simulink model "bldc"  (R2022a)
settings: Solver=VariableStepAuto  StartTime=0.0  StopTime=60  FixedStep=0.0001  MaxStep=0.01  RelTol=1e-3
model workspace (MAT data in the model file):
  gPWM_U_ptr : handle (value not decoded)
  gPWM_V_ptr : handle (value not decoded)
  gPWM_W_ptr : handle (value not decoded)
values from neighbouring files (symbols this model uses):
  D = 0.00075    [init_bldc.m]
  J = 0.00025    [init_bldc.m]
  Ld = 0.0009447    [init_bldc.m]
  Lq = 0.0009447    [init_bldc.m]
  P = 7    [init_bldc.m]
  qsi = 0.006198    [init_bldc.m]
  R = 0.453    [init_bldc.m]
  V = 24    [init_bldc.m]
settings Model: Creator=sshio  LastModifiedBy=sshio
settings DebuggingCC: UnconnectedInputMsg=warning  UnconnectedOutputMsg=warning  UnconnectedLineMsg=warning
settings RTWCC: DLArmComputeVersion=19.05

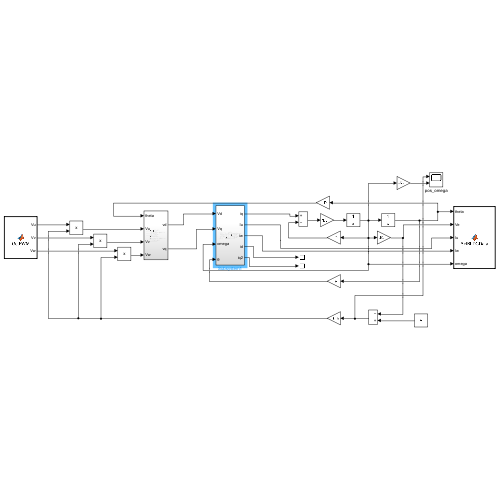
[thumbnail: Simulink's stored preview of the top-level diagram]
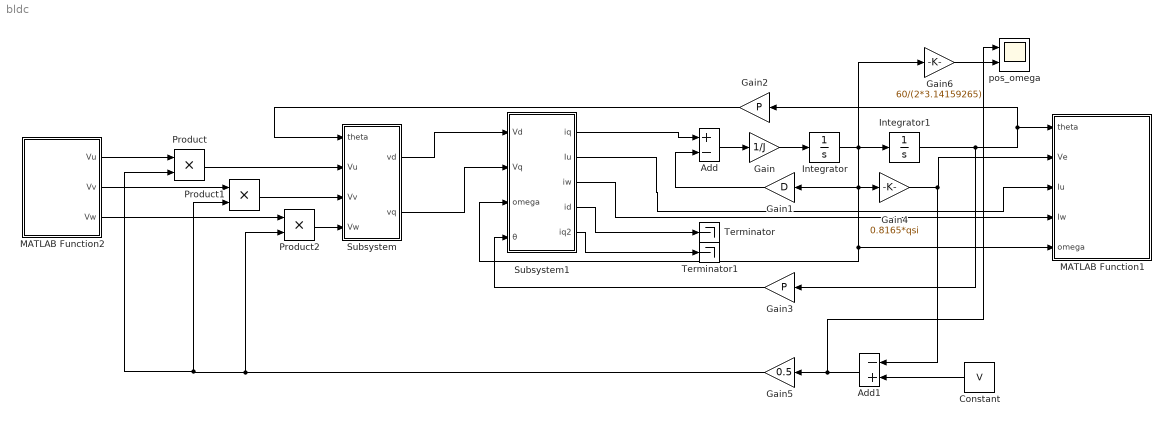
== system bldc ==
  Add : Sum  Inputs=+-
  Add1 : Sum  Inputs=-+
  Constant : Constant  Value=V
  Gain : Gain  Gain=1/J
  Gain1 : Gain  Gain=D
  Gain2 : Gain  Gain=P
  Gain3 : Gain  Gain=P
  Gain4 : Gain  Gain=0.8165*qsi
  Gain5 : Gain  Gain=0.5
  Gain6 : Gain  Gain=60/(2*3.14159265)
  Integrator : Integrator
  Integrator1 : Integrator
  MATLAB Function1 : MATLAB Function  TreatAsAtomicUnit=on  SystemSampleTime=0.0001
  MATLAB Function2 : MATLAB Function  TreatAsAtomicUnit=on  SystemSampleTime=0.0001
  Product : Product
  Product1 : Product
  Product2 : Product
  Subsystem : Subsystem
  Subsystem1 : Subsystem
  Terminator : Terminator
  Terminator1 : Terminator
  pos_omega : Scope  NumInputPorts=2
  wires:
  Subsystem/2(vq) -> Subsystem1/2(Vq)
  Integrator/1 -> Gain6/1, Integrator1/1, Gain4/1, Gain1/1, MATLAB Function1/5(omega), Subsystem1/3(omega)
  Gain/1 -> Integrator/1
  Add/1 -> Gain/1
  Subsystem1/1(iq) -> Add/1
  Gain1/1 -> Add/2
  Gain2/1 -> Subsystem/1(theta)
  Gain3/1 -> Subsystem1/4(θ)
  Subsystem1/3(iw) -> MATLAB Function1/4(Iw)
  Gain4/1 -> Add1/1, MATLAB Function1/2(Ve)
  Constant/1 -> Add1/2
  Gain5/1 -> Product/2, Product1/2, Product2/2
  Product2/1 -> Subsystem/4(Vw)
  MATLAB Function2/2(Vv) -> Product1/1
  MATLAB Function2/3(Vw) -> Product2/1
  Product1/1 -> Subsystem/3(Vv)
  Product/1 -> Subsystem/2(Vu)
  MATLAB Function2/1(Vu) -> Product/1
  Integrator1/1 -> Gain3/1, Gain2/1, MATLAB Function1/1(theta)
  Subsystem1/2(Iu) -> MATLAB Function1/3(Iu)
  Add1/1 -> pos_omega/1, Gain5/1
  Gain6/1 -> pos_omega/2
  Subsystem/1(vd) -> Subsystem1/1(Vd)
  Subsystem1/4(id) -> Terminator/1
  Subsystem1/5(iq2) -> Terminator1/1

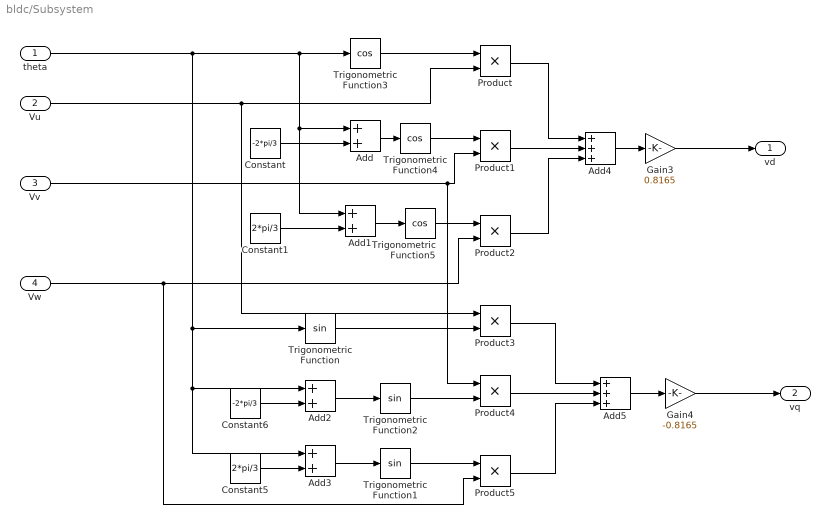
== system bldc/Subsystem ==
  theta : Inport
  Vu : Inport  Port=2
  Vv : Inport  Port=3
  Vw : Inport  Port=4
  Add{,1..3} (4 alike) : Sum
  Add4 : Sum  Inputs=+++
  Add5 : Sum  Inputs=+++
  Constant : Constant  Value=-2*pi/3
  Constant1 : Constant  Value=2*pi/3
  Constant5 : Constant  Value=2*pi/3
  Constant6 : Constant  Value=-2*pi/3
  Gain3 : Gain  Gain=0.8165
  Gain4 : Gain  Gain=-0.8165
  Product{,1..5} (6 alike) : Product
  Trigonometric Function : Trigonometry
  Trigonometric Function1 : Trigonometry
  Trigonometric Function2 : Trigonometry
  Trigonometric Function3 : Trigonometry  Operator=cos
  Trigonometric Function4 : Trigonometry  Operator=cos
  Trigonometric Function5 : Trigonometry  Operator=cos
  vd : Outport
  vq : Outport  Port=2
  wires:
  Product2/1 -> Add4/3
  theta/1 -> Add3/1, Add2/1, Trigonometric Function/1, Add1/1, Add/1, Trigonometric Function3/1
  Add4/1 -> Gain3/1
  Trigonometric Function3/1 -> Product/1
  Trigonometric Function5/1 -> Product2/1
  Add/1 -> Trigonometric Function4/1
  Product1/1 -> Add4/2
  Trigonometric Function/1 -> Product3/2
  Constant/1 -> Add/2
  Vu/1 -> Product/2, Product3/1
  Add1/1 -> Trigonometric Function5/1
  Trigonometric Function4/1 -> Product1/1
  Vv/1 -> Product4/1, Product1/2
  Add2/1 -> Trigonometric Function2/1
  Constant6/1 -> Add2/2
  Constant5/1 -> Add3/2
  Add3/1 -> Trigonometric Function1/1
  Trigonometric Function2/1 -> Product4/2
  Trigonometric Function1/1 -> Product5/1
  Constant1/1 -> Add1/2
  Product4/1 -> Add5/2
  Vw/1 -> Product2/2, Product5/2
  Product3/1 -> Add5/1
  Gain4/1 -> vq/1
  Add5/1 -> Gain4/1
  Product/1 -> Add4/1
  Product5/1 -> Add5/3
  Gain3/1 -> vd/1

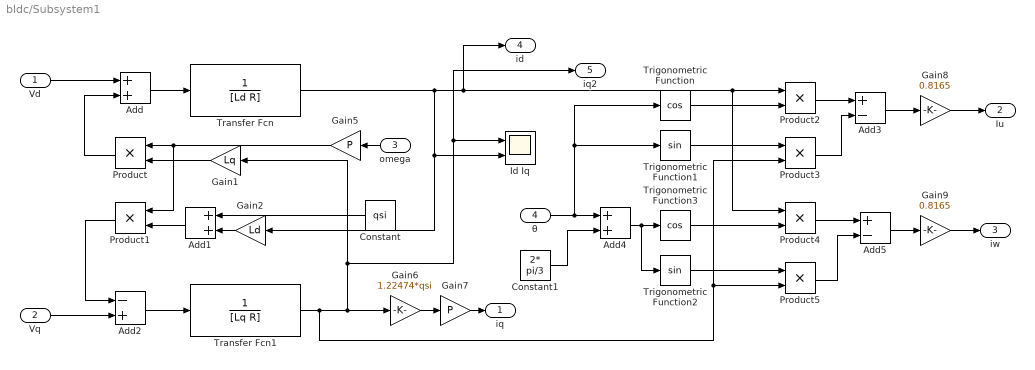
== system bldc/Subsystem1 ==
  Vd : Inport
  Vq : Inport  Port=2
  omega : Inport  Port=3
  θ : Inport  Port=4
  Add : Sum
  Add1 : Sum
  Add2 : Sum  Inputs=-+
  Add3 : Sum  Inputs=+-
  Add4 : Sum
  Add5 : Sum  Inputs=+-
  Constant : Constant  Value=qsi
  Constant1 : Constant  Value=2* pi/3
  Gain1 : Gain  Gain=Lq
  Gain2 : Gain  Gain=Ld
  Gain5 : Gain  Gain=P
  Gain6 : Gain  Gain=1.22474*qsi
  Gain7 : Gain  Gain=P
  Gain8 : Gain  Gain=0.8165
  Gain9 : Gain  Gain=0.8165
  Id Iq : Scope  NumInputPorts=2
  Product{,1..5} (6 alike) : Product
  Transfer Fcn : TransferFcn  Denominator=[Ld R]
  Transfer Fcn1 : TransferFcn  Denominator=[Lq R]
  Trigonometric Function : Trigonometry  Operator=cos
  Trigonometric Function1 : Trigonometry
  Trigonometric Function2 : Trigonometry
  Trigonometric Function3 : Trigonometry  Operator=cos
  iq : Outport
  Iu : Outport  Port=2
  iw : Outport  Port=3
  id : Outport  Port=4
  iq2 : Outport  Port=5
  wires:
  Product1/1 -> Add2/1
  Gain7/1 -> iq/1
  Gain5/1 -> Product/1, Product1/1
  Gain1/1 -> Product/2
  Constant/1 -> Add1/1
  Add2/1 -> Transfer Fcn1/1
  Add/1 -> Transfer Fcn/1
  Product/1 -> Add/2
  Gain2/1 -> Add1/2
  Add1/1 -> Product1/2
  Gain6/1 -> Gain7/1
  Vq/1 -> Add2/2
  omega/1 -> Gain5/1
  Vd/1 -> Add/1
  θ/1 -> Add4/1, Trigonometric Function1/1, Trigonometric Function/1
  Trigonometric Function/1 -> Product2/2
  Trigonometric Function1/1 -> Product3/1
  Product2/1 -> Add3/1
  Product3/1 -> Add3/2
  Add3/1 -> Gain8/1
  Gain8/1 -> Iu/1
  Constant1/1 -> Add4/2
  Add4/1 -> Trigonometric Function2/1, Trigonometric Function3/1
  Trigonometric Function3/1 -> Product4/2
  Trigonometric Function2/1 -> Product5/1
  Product4/1 -> Add5/1
  Product5/1 -> Add5/2
  Add5/1 -> Gain9/1
  Gain9/1 -> iw/1
  Transfer Fcn1/1 -> Product5/2, Product3/2, Gain6/1, Id Iq/1, iq2/1, Gain1/1
  Transfer Fcn/1 -> id/1, Product4/1, Product2/1, Gain2/1, Id Iq/2

== matlab function bldc/MATLAB Function1 ==
  data: theta input; Ve input; Iu input; Iw input; omega input
function SetBLDCData(theta, Ve, Iu, Iw, omega)
    coder.extrinsic('MatSetBLDCData');
    coder.extrinsic('MatReqInt_BLDC');
    MatSetBLDCData(theta, Ve, Iu, Iw, omega);
    MatReqInt_BLDC();
end

== matlab function bldc/MATLAB Function2 ==
  data: Vu output; Vv output; Vw output
function [Vu,Vv,Vw] = GetPWM()
    coder.extrinsic('MatGetBLDC_PWM_U');
    coder.extrinsic('MatGetBLDC_PWM_V');
    coder.extrinsic('MatGetBLDC_PWM_W');
    Vu = 0.0;
    Vv = 0.0;
    Vw = 0.0;
    Vu = MatGetBLDC_PWM_U();
    Vv = MatGetBLDC_PWM_V();
    Vw = MatGetBLDC_PWM_W();
%       Vu = 12;
%       Vv = 0;
%       Vw = -12;
end
